simulink model "HW7_v1"  (R2019b)
settings: Solver=VariableStepAuto  StartTime=0.0  StopTime=30  RelTol=1e-3
values from neighbouring files (symbols this model uses):
  A1 = [0 1;        0 0]    [HW7.m]
  A1_wiener = [0 1 ;               0 0]    [HW7.m]
  B1 = [0;      -0.067]    [HW7.m]
  B1_wiener = [0;               1]    [HW7.m]
  C1 = [1 0;       0 1;      -1 0 ;        0 0]    [HW7.m]
  C1_wiener = [1 0]    [HW7.m]
  D1 = [0 ... (first row only)    [HW7.m]
  D1_wiener = [0]    [HW7.m]
  K1 = lqr(A1, B1, Q1, R1)    [HW7.m]
  L1 = lqe(A1_cont, G1, C1_cont, Q1, R1, N1)    [HW7.m]
  M_inv = inv(M_motor)    [HW7.m]
  M_motor = [1, 1, 1, -1;             1, 1, -1, 1;             1, -1, -1, -1;             1, -1, 1, 1 ]    [HW7.m]
  tau2 = 0.015915    [HW7.m]
  V = 5    [HW7.m]
  V0 = 5    [HW7.m]
undefined symbols (not defined in the file or in its folder): DiscIntNeverNeededParam
settings Model: Creator=cwhipp  LastModifiedBy=cwhipp

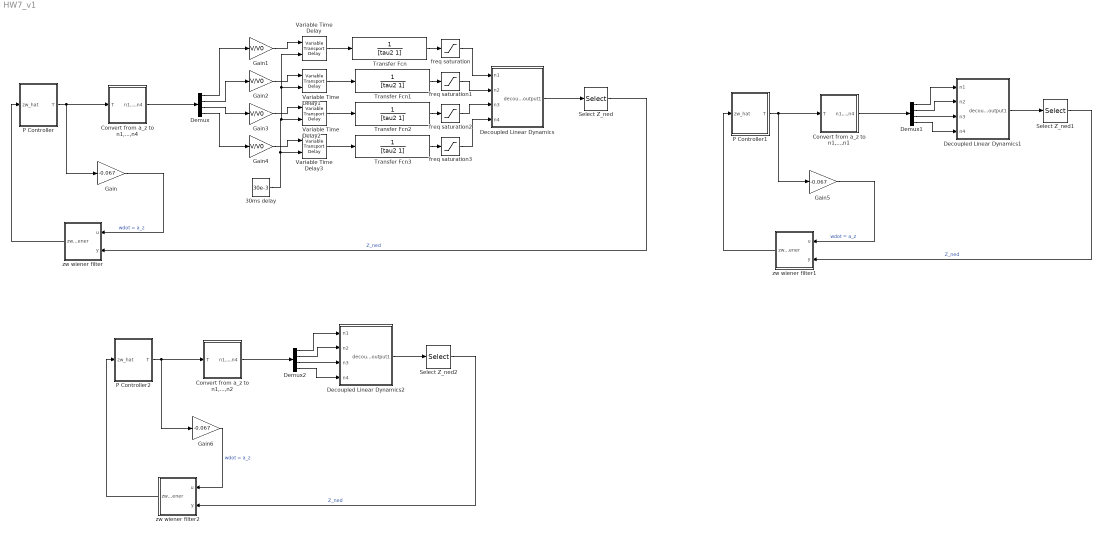
== system HW7_v1 ==
  30ms delay : Constant  Value=30e-3
  Convert from a_z to n1,...,n1 : Subsystem
  Convert from a_z to n1,...,n2 : Subsystem
  Convert from a_z to n1,...,n4 : Subsystem
  Decoupled Linear Dynamics : Subsystem
  Decoupled Linear Dynamics1 : Subsystem
  Decoupled Linear Dynamics2 : Subsystem
  Demux : Demux
  Demux1 : Demux
  Demux2 : Demux
  Gain : Gain  Gain=-0.067
  Gain{1..4} (4 alike) : Gain  Gain=V/V0
  Gain5 : Gain  Gain=-0.067
  Gain6 : Gain  Gain=-0.067
  P Controller : Subsystem
  P Controller1 : Subsystem
  P Controller2 : Subsystem
  Select Z_ned : Selector  InputPortWidth=4  IndexOptions=Index vector (dialog)  Indices=[1]  OutputSizes=1
  Select Z_ned1 : Selector  InputPortWidth=4  IndexOptions=Index vector (dialog)  Indices=[1]  OutputSizes=1
  Select Z_ned2 : Selector  InputPortWidth=4  IndexOptions=Index vector (dialog)  Indices=[1]  OutputSizes=1
  Transfer Fcn{,1..3} (4 alike) : TransferFcn  Denominator=[tau2 1]
  Variable Time Delay{,1..3} (4 alike) : VariableTransportDelay  MaximumDelay=10
  freq saturation{,1..3} (4 alike) : Saturate  UpperLimit=500  LowerLimit=10
  zw wiener filter : Subsystem
  zw wiener filter1 : Subsystem
  zw wiener filter2 : Subsystem
  wires:
  Decoupled Linear Dynamics/1(decoupoutput1) -> Select Z_ned/1
  Select Z_ned/1 -> zw wiener filter/2(y)  "Z_ned"
  zw wiener filter/1(zw_wiener) -> P Controller/1(zw_hat)
  P Controller/1(T) -> Convert from a_z to n1,...,n4/1(T), Gain/1
  Gain/1 -> zw wiener filter/1(u)  "wdot = a_z"
  Convert from a_z to n1,...,n4/1(n1,...,n4) -> Demux/1
  Transfer Fcn1/1 -> freq saturation1/1
  Transfer Fcn/1 -> freq saturation/1
  Transfer Fcn2/1 -> freq saturation2/1
  Transfer Fcn3/1 -> freq saturation3/1
  Demux/1 -> Gain1/1
  Demux/2 -> Gain2/1
  Demux/3 -> Gain3/1
  Demux/4 -> Gain4/1
  freq saturation/1 -> Decoupled Linear Dynamics/1(n1)
  freq saturation1/1 -> Decoupled Linear Dynamics/2(n2)
  freq saturation2/1 -> Decoupled Linear Dynamics/3(n3)
  freq saturation3/1 -> Decoupled Linear Dynamics/4(n4)
  Gain4/1 -> Variable Time Delay3/1
  Gain3/1 -> Variable Time Delay2/1
  Gain2/1 -> Variable Time Delay1/1
  Gain1/1 -> Variable Time Delay/1
  Variable Time Delay/1 -> Transfer Fcn/1
  Variable Time Delay1/1 -> Transfer Fcn1/1
  Variable Time Delay2/1 -> Transfer Fcn2/1
  Variable Time Delay3/1 -> Transfer Fcn3/1
  30ms delay/1 -> Variable Time Delay3/2, Variable Time Delay/2, Variable Time Delay1/2, Variable Time Delay2/2
  Gain5/1 -> zw wiener filter1/1(u)  "wdot = a_z"
  zw wiener filter1/1(zw_wiener) -> P Controller1/1(zw_hat)
  Select Z_ned1/1 -> zw wiener filter1/2(y)  "Z_ned"
  Decoupled Linear Dynamics1/1(decoupoutput1) -> Select Z_ned1/1
  Convert from a_z to n1,...,n1/1(n1,...,n4) -> Demux1/1
  Demux1/4 -> Decoupled Linear Dynamics1/4(n4)
  Demux1/1 -> Decoupled Linear Dynamics1/1(n1)
  P Controller1/1(T) -> Convert from a_z to n1,...,n1/1(T), Gain5/1
  Demux1/3 -> Decoupled Linear Dynamics1/3(n3)
  Demux1/2 -> Decoupled Linear Dynamics1/2(n2)
  Demux2/1 -> Decoupled Linear Dynamics2/1(n1)
  Demux2/2 -> Decoupled Linear Dynamics2/2(n2)
  Convert from a_z to n1,...,n2/1(n1,...,n4) -> Demux2/1
  Select Z_ned2/1 -> zw wiener filter2/2(y)  "Z_ned"
  Decoupled Linear Dynamics2/1(decoupoutput1) -> Select Z_ned2/1
  P Controller2/1(T) -> Convert from a_z to n1,...,n2/1(T), Gain6/1
  Gain6/1 -> zw wiener filter2/1(u)  "wdot = a_z"
  zw wiener filter2/1(zw_wiener) -> P Controller2/1(zw_hat)
  Demux2/4 -> Decoupled Linear Dynamics2/4(n4)
  Demux2/3 -> Decoupled Linear Dynamics2/3(n3)

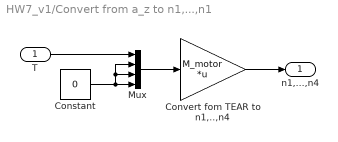
== system HW7_v1/Convert from a_z to n1,...,n1 ==
  T : Inport
  Constant : Constant  Value=0
  Convert fom TEAR to n1,..,n4 : Gain  Gain=M_motor  Multiplication=Matrix(K*u)
  Mux : Mux
  n1,...,n4 : Outport
  wires:
  Constant/1 -> Mux/4, Mux/3, Mux/2
  Convert fom TEAR to n1,..,n4/1 -> n1,...,n4/1
  Mux/1 -> Convert fom TEAR to n1,..,n4/1
  T/1 -> Mux/1

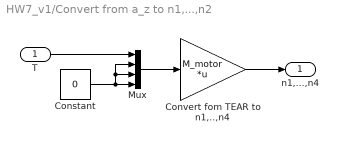
== system HW7_v1/Convert from a_z to n1,...,n2 ==
  T : Inport
  Constant : Constant  Value=0
  Convert fom TEAR to n1,..,n4 : Gain  Gain=M_motor  Multiplication=Matrix(K*u)
  Mux : Mux
  n1,...,n4 : Outport
  wires:
  Constant/1 -> Mux/4, Mux/3, Mux/2
  Convert fom TEAR to n1,..,n4/1 -> n1,...,n4/1
  Mux/1 -> Convert fom TEAR to n1,..,n4/1
  T/1 -> Mux/1

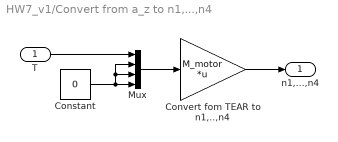
== system HW7_v1/Convert from a_z to n1,...,n4 ==
  T : Inport
  Constant : Constant  Value=0
  Convert fom TEAR to n1,..,n4 : Gain  Gain=M_motor  Multiplication=Matrix(K*u)
  Mux : Mux
  n1,...,n4 : Outport
  wires:
  Constant/1 -> Mux/4, Mux/3, Mux/2
  Convert fom TEAR to n1,..,n4/1 -> n1,...,n4/1
  Mux/1 -> Convert fom TEAR to n1,..,n4/1
  T/1 -> Mux/1

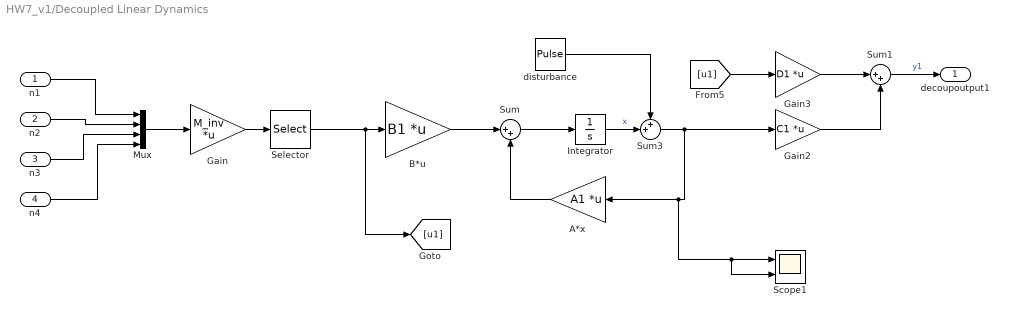
== system HW7_v1/Decoupled Linear Dynamics ==
  n1 : Inport
  n2 : Inport  Port=2
  n3 : Inport  Port=3
  n4 : Inport  Port=4
  A*x : Gain  Gain=A1  Multiplication=Matrix(K*u)
  B*u : Gain  Gain=B1  Multiplication=Matrix(K*u)
  Gain : Gain  Gain=M_inv  Multiplication=Matrix(K*u)
  Gain2 : Gain  Gain=C1  Multiplication=Matrix(K*u)
  Gain3 : Gain  Gain=D1  Multiplication=Matrix(K*u)
  Integrator : Integrator
  Mux : Mux
  Scope1 : Scope  NumInputPorts=2
  Selector : Selector  InputPortWidth=4  IndexOptions=Index vector (dialog)  Indices=1  OutputSizes=1
  Sum : Sum  Inputs=|++
  Sum1 : Sum  Inputs=|++
  Sum3 : Sum  Inputs=++|
  "disturbance " : DiscretePulseGenerator  PulseType=Time based  Period=40  PulseWidth=2.5
  decoupoutput1 : Outport
  wires:
  Sum/1 -> Integrator/1
  A*x/1 -> Sum/2
  Gain3/1 -> Sum1/1
  Sum1/1 -> decoupoutput1/1  "y1"
  B*u/1 -> Sum/1
  Gain2/1 -> Sum1/2
  [u1] -> Gain3/1
  n1/1 -> Mux/1
  n2/1 -> Mux/2
  n3/1 -> Mux/3
  n4/1 -> Mux/4
  Mux/1 -> Gain/1
  Gain/1 -> Selector/1
  Selector/1 -> [u1], B*u/1
  "disturbance "/1 -> Sum3/1
  Integrator/1 -> Sum3/2  "x"
  Sum3/1 -> Gain2/1, Scope1/2, Scope1/1, A*x/1

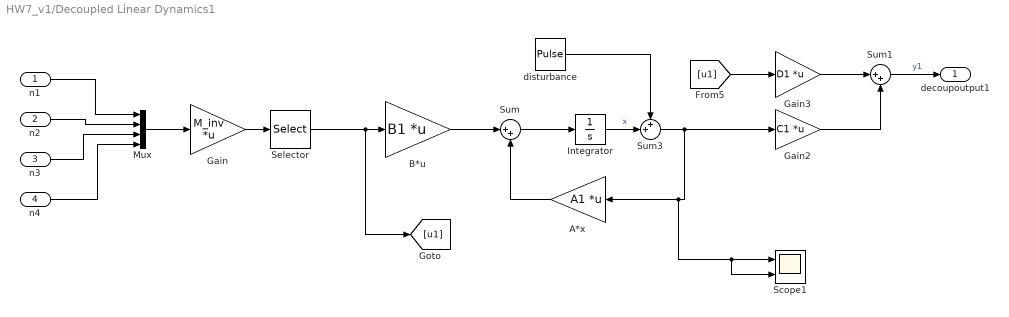
== system HW7_v1/Decoupled Linear Dynamics1 ==
  n1 : Inport
  n2 : Inport  Port=2
  n3 : Inport  Port=3
  n4 : Inport  Port=4
  A*x : Gain  Gain=A1  Multiplication=Matrix(K*u)
  B*u : Gain  Gain=B1  Multiplication=Matrix(K*u)
  Gain : Gain  Gain=M_inv  Multiplication=Matrix(K*u)
  Gain2 : Gain  Gain=C1  Multiplication=Matrix(K*u)
  Gain3 : Gain  Gain=D1  Multiplication=Matrix(K*u)
  Integrator : Integrator
  Mux : Mux
  Scope1 : Scope  NumInputPorts=2
  Selector : Selector  InputPortWidth=4  IndexOptions=Index vector (dialog)  Indices=1  OutputSizes=1
  Sum : Sum  Inputs=|++
  Sum1 : Sum  Inputs=|++
  Sum3 : Sum  Inputs=++|
  "disturbance " : DiscretePulseGenerator  PulseType=Time based  Period=40  PulseWidth=2.5
  decoupoutput1 : Outport
  wires:
  Sum/1 -> Integrator/1
  A*x/1 -> Sum/2
  Gain3/1 -> Sum1/1
  Sum1/1 -> decoupoutput1/1  "y1"
  B*u/1 -> Sum/1
  Gain2/1 -> Sum1/2
  [u1] -> Gain3/1
  n1/1 -> Mux/1
  n2/1 -> Mux/2
  n3/1 -> Mux/3
  n4/1 -> Mux/4
  Mux/1 -> Gain/1
  Gain/1 -> Selector/1
  Selector/1 -> [u1], B*u/1
  "disturbance "/1 -> Sum3/1
  Integrator/1 -> Sum3/2  "x"
  Sum3/1 -> Gain2/1, Scope1/2, Scope1/1, A*x/1

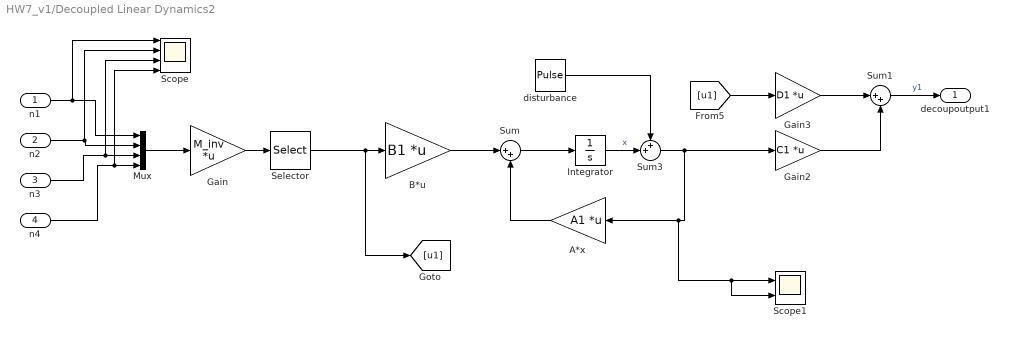
== system HW7_v1/Decoupled Linear Dynamics2 ==
  n1 : Inport
  n2 : Inport  Port=2
  n3 : Inport  Port=3
  n4 : Inport  Port=4
  A*x : Gain  Gain=A1  Multiplication=Matrix(K*u)
  B*u : Gain  Gain=B1  Multiplication=Matrix(K*u)
  Gain : Gain  Gain=M_inv  Multiplication=Matrix(K*u)
  Gain2 : Gain  Gain=C1  Multiplication=Matrix(K*u)
  Gain3 : Gain  Gain=D1  Multiplication=Matrix(K*u)
  Integrator : Integrator
  Mux : Mux
  Scope : Scope  NumInputPorts=4
  Scope1 : Scope  NumInputPorts=2
  Selector : Selector  InputPortWidth=4  IndexOptions=Index vector (dialog)  Indices=1  OutputSizes=1
  Sum : Sum  Inputs=|++
  Sum1 : Sum  Inputs=|++
  Sum3 : Sum  Inputs=++|
  "disturbance " : DiscretePulseGenerator  PulseType=Time based  Period=40  PulseWidth=2.5
  decoupoutput1 : Outport
  wires:
  Sum/1 -> Integrator/1
  A*x/1 -> Sum/2
  Gain3/1 -> Sum1/1
  Sum1/1 -> decoupoutput1/1  "y1"
  B*u/1 -> Sum/1
  Gain2/1 -> Sum1/2
  [u1] -> Gain3/1
  n1/1 -> Mux/1, Scope/1
  n2/1 -> Mux/2, Scope/2
  n3/1 -> Scope/3, Mux/3
  n4/1 -> Scope/4, Mux/4
  Mux/1 -> Gain/1
  Gain/1 -> Selector/1
  Selector/1 -> [u1], B*u/1
  "disturbance "/1 -> Sum3/1
  Integrator/1 -> Sum3/2  "x"
  Sum3/1 -> Gain2/1, Scope1/2, Scope1/1, A*x/1

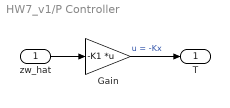
== system HW7_v1/P Controller ==
  zw_hat : Inport
  Gain : Gain  Gain=-K1  Multiplication=Matrix(K*u)
  T : Outport
  wires:
  Gain/1 -> T/1  "u = -Kx"
  zw_hat/1 -> Gain/1

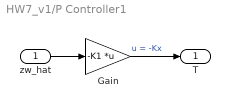
== system HW7_v1/P Controller1 ==
  zw_hat : Inport
  Gain : Gain  Gain=-K1  Multiplication=Matrix(K*u)
  T : Outport
  wires:
  Gain/1 -> T/1  "u = -Kx"
  zw_hat/1 -> Gain/1

== system HW7_v1/P Controller2 ==
  zw_hat : Inport
  Gain : Gain  Gain=-K1  Multiplication=Matrix(K*u)
  T : Outport
  wires:
  Gain/1 -> T/1  "u = -Kx"
  zw_hat/1 -> Gain/1

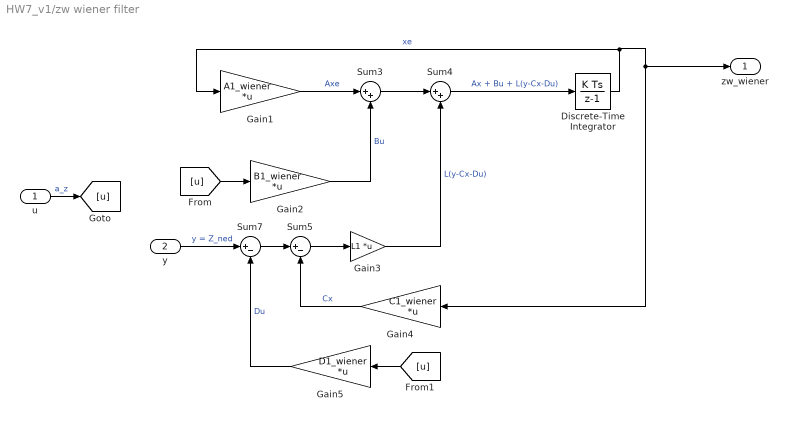
== system HW7_v1/zw wiener filter ==
  u : Inport
  y : Inport  Port=2
  Discrete-Time Integrator : DiscreteIntegrator  SampleTime=-1  ICPrevOutput=DiscIntNeverNeededParam  ICPrevScaledInput=DiscIntNeverNeededParam
  Gain1 : Gain  Gain=A1_wiener  Multiplication=Matrix(K*u)
  Gain2 : Gain  Gain=B1_wiener  Multiplication=Matrix(K*u)
  Gain3 : Gain  Gain=L1  Multiplication=Matrix(K*u)
  Gain4 : Gain  Gain=C1_wiener  Multiplication=Matrix(K*u)
  Gain5 : Gain  Gain=D1_wiener  Multiplication=Matrix(K*u)
  Sum3 : Sum  Inputs=|++
  Sum4 : Sum  Inputs=|++
  Sum5 : Sum  Inputs=|+-
  Sum7 : Sum  Inputs=|+-
  zw_wiener : Outport
  wires:
  y/1 -> Sum7/1  "y = Z_ned"
  Gain3/1 -> Sum4/2  "L(y-Cx-Du)"
  Gain1/1 -> Sum3/1  "Axe"
  Sum4/1 -> Discrete-Time Integrator/1  "Ax + Bu + L(y-Cx-Du)"
  Discrete-Time Integrator/1 -> Gain4/1, zw_wiener/1, Gain1/1  "xe"
  Gain4/1 -> Sum5/2  "Cx"
  Gain2/1 -> Sum3/2  "Bu"
  Sum5/1 -> Gain3/1
  Sum7/1 -> Sum5/1
  Sum3/1 -> Sum4/1
  Gain5/1 -> Sum7/2  "Du"
  u/1 -> [u]  "a_z"
  [u] -> Gain2/1
  [u] -> Gain5/1

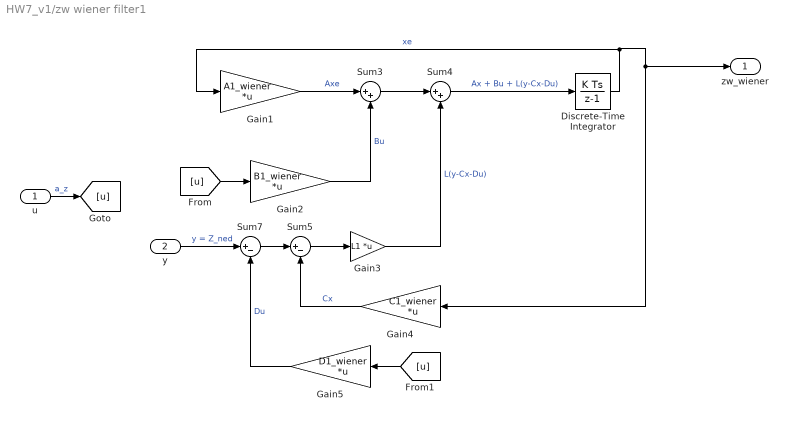
== system HW7_v1/zw wiener filter1 ==
  u : Inport
  y : Inport  Port=2
  Discrete-Time Integrator : DiscreteIntegrator  SampleTime=-1  ICPrevOutput=DiscIntNeverNeededParam  ICPrevScaledInput=DiscIntNeverNeededParam
  Gain1 : Gain  Gain=A1_wiener  Multiplication=Matrix(K*u)
  Gain2 : Gain  Gain=B1_wiener  Multiplication=Matrix(K*u)
  Gain3 : Gain  Gain=L1  Multiplication=Matrix(K*u)
  Gain4 : Gain  Gain=C1_wiener  Multiplication=Matrix(K*u)
  Gain5 : Gain  Gain=D1_wiener  Multiplication=Matrix(K*u)
  Sum3 : Sum  Inputs=|++
  Sum4 : Sum  Inputs=|++
  Sum5 : Sum  Inputs=|+-
  Sum7 : Sum  Inputs=|+-
  zw_wiener : Outport
  wires:
  y/1 -> Sum7/1  "y = Z_ned"
  Gain3/1 -> Sum4/2  "L(y-Cx-Du)"
  Gain1/1 -> Sum3/1  "Axe"
  Sum4/1 -> Discrete-Time Integrator/1  "Ax + Bu + L(y-Cx-Du)"
  Discrete-Time Integrator/1 -> Gain4/1, zw_wiener/1, Gain1/1  "xe"
  Gain4/1 -> Sum5/2  "Cx"
  Gain2/1 -> Sum3/2  "Bu"
  Sum5/1 -> Gain3/1
  Sum7/1 -> Sum5/1
  Sum3/1 -> Sum4/1
  Gain5/1 -> Sum7/2  "Du"
  u/1 -> [u]  "a_z"
  [u] -> Gain2/1
  [u] -> Gain5/1

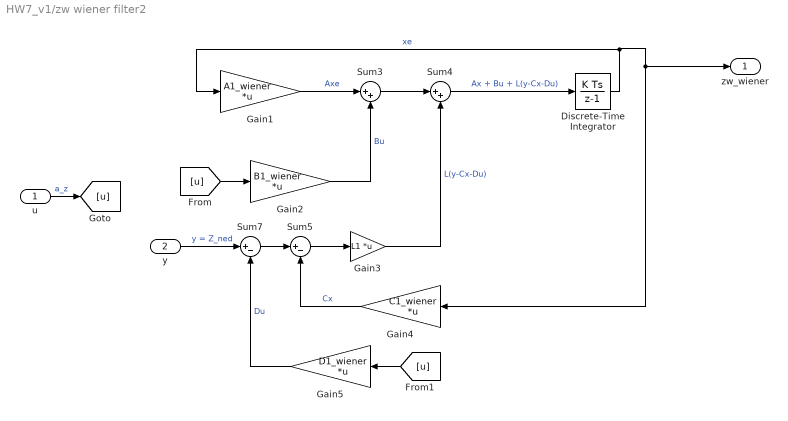
== system HW7_v1/zw wiener filter2 ==
  u : Inport
  y : Inport  Port=2
  Discrete-Time Integrator : DiscreteIntegrator  SampleTime=-1  ICPrevOutput=DiscIntNeverNeededParam  ICPrevScaledInput=DiscIntNeverNeededParam
  Gain1 : Gain  Gain=A1_wiener  Multiplication=Matrix(K*u)
  Gain2 : Gain  Gain=B1_wiener  Multiplication=Matrix(K*u)
  Gain3 : Gain  Gain=L1  Multiplication=Matrix(K*u)
  Gain4 : Gain  Gain=C1_wiener  Multiplication=Matrix(K*u)
  Gain5 : Gain  Gain=D1_wiener  Multiplication=Matrix(K*u)
  Sum3 : Sum  Inputs=|++
  Sum4 : Sum  Inputs=|++
  Sum5 : Sum  Inputs=|+-
  Sum7 : Sum  Inputs=|+-
  zw_wiener : Outport
  wires:
  y/1 -> Sum7/1  "y = Z_ned"
  Gain3/1 -> Sum4/2  "L(y-Cx-Du)"
  Gain1/1 -> Sum3/1  "Axe"
  Sum4/1 -> Discrete-Time Integrator/1  "Ax + Bu + L(y-Cx-Du)"
  Discrete-Time Integrator/1 -> Gain4/1, zw_wiener/1, Gain1/1  "xe"
  Gain4/1 -> Sum5/2  "Cx"
  Gain2/1 -> Sum3/2  "Bu"
  Sum5/1 -> Gain3/1
  Sum7/1 -> Sum5/1
  Sum3/1 -> Sum4/1
  Gain5/1 -> Sum7/2  "Du"
  u/1 -> [u]  "a_z"
  [u] -> Gain2/1
  [u] -> Gain5/1
